simulink library "Lib_Vol_FlowChar_TMATS_org"  (Simulink 10.0)
settings: Solver=ode45  StartTime=0.0  StopTime=10.0  RelTol=1e-3  EnableMultiTasking=on
Description:
  | Thomas Modules
settings Model: Creator=jwchapm2  LastModifiedBy=bhisma

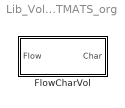
== system Lib_Vol_FlowChar_TMATS_org ==
  FlowCharVol : Subsystem

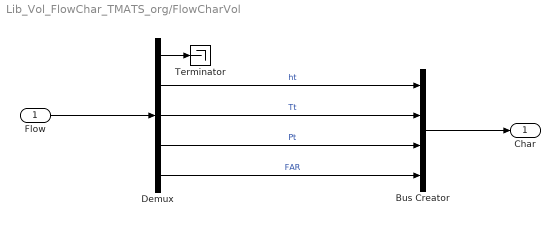
== system Lib_Vol_FlowChar_TMATS_org/FlowCharVol ==
  Flow : Inport
  Bus Creator : BusCreator  Inputs=4
  Demux : Demux  Outputs=5
  Terminator : Terminator
  Char : Outport
  wires:
  Bus Creator/1 -> Char/1
  Flow/1 -> Demux/1
  Demux/4 -> Bus Creator/3  "Pt"
  Demux/3 -> Bus Creator/2  "Tt"
  Demux/2 -> Bus Creator/1  "ht"
  Demux/5 -> Bus Creator/4  "FAR"
  Demux/1 -> Terminator/1
